simulink model "positionAlignment"  (R2019b)
settings: Solver=FixedStepAuto  StartTime=tStart  StopTime=tEnd  FixedStep=tStep  RelTol=1e-3
values from neighbouring files (symbols this model uses):
  headingCurrent = headings(ind)    [simulation.m]
  headingPrevious = -headingCurrent    [simulation.m]
  pathLength = sqrt((XYCurrent(1)-XYPrevious(1))^2 + (XYCurrent(2)-XYPrevious(2))^2)    [simulation.m]
  tStep = 0.01    [simulation.m]
  X = (1:imWidth)/imWidth*yardWidth    [getTerrainBinary1.m]
  XYCurrent = wayPointsXY(ind+1,:)    [simulation.m]
  XYPrevious = XYCurrent    [simulation.m]
  Y = (1:imHeight)/imHeight*yardHeight    [getTerrainBinary1.m]
  Z = double(yardBright)/255*height    [createVirtualWorld.m]    (also in getTerrainBinary1.m = image; getTerrainBinary2.m = image; simulation.m = (sin(4*Y))/8; terrainMain.m = getTerrainBinary2(height, yardWidth, yardHeight, yardBright,)
libraries: simulink x1
settings Model: Creator=sebas  LastModifiedBy=sebas

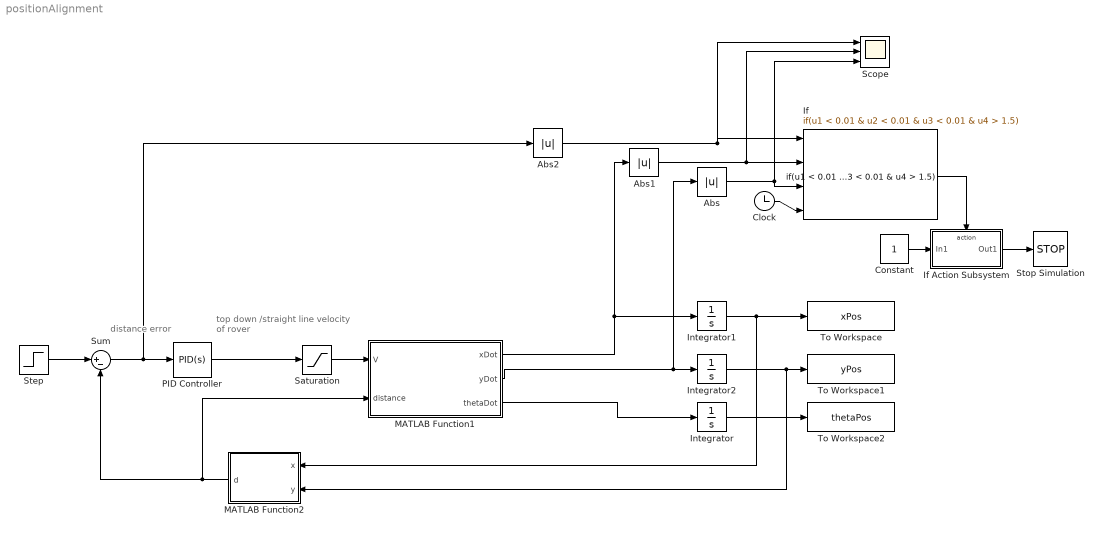
== system positionAlignment ==
  note: top down /straight line
      | velocity of rover
  note: distance error
  Abs : Abs
  Abs1 : Abs
  Abs2 : Abs
  Clock : Clock
  Constant : Constant
  If : If  NumInputs=4  IfExpression=u1 < 0.01 & u2 < 0.01 & u3 < 0.01 & u4 > 1.5  ShowElse=off
  If Action Subsystem : Subsystem  TreatAsAtomicUnit=on
  Integrator : Integrator  InitialCondition=headingPrevious
  Integrator1 : Integrator
  Integrator2 : Integrator
  MATLAB Function1 : MATLAB Function  TreatAsAtomicUnit=on
  MATLAB Function2 : MATLAB Function  TreatAsAtomicUnit=on
  PID Controller : simulink/Continuous/PID Controller  Controller=PID  Form=Parallel  TimeDomain=Continuous-time  SampleTime=-1  IntegratorMethod=Forward Euler  FilterMethod=Forward Euler  ControllerParametersSource=internal  P=0.31  I=0.0004396  D=-0.0175  UseFilter=on  N=18.11  TunerSelectOption=Transfer Function Based (PID Tuner App)  InitialConditionSource=internal  InitialConditionForIntegrator=0  InitialConditionForFilter=0  DifferentiatorICPrevScaledInput=0  ExternalReset=none  TrackingMode=off  Kt=1  LimitOutput=off  UpperSaturationLimit=inf  LowerSaturationLimit=-inf  LinearizeAsGain=on  AntiWindupMode=none  Kb=1  POutMin=[]  POutMax=[]  IOutMin=[]  IOutMax=[]  DOutMin=[]  DOutMax=[]  NOutMin=[]  NOutMax=[]  SumOutMin=[]  SumOutMax=[]  SaturationOutMin=[]  SaturationOutMax=[]  PParamMin=[]  PParamMax=[]  IParamMin=[]  IParamMax=[]  DParamMin=[]  DParamMax=[]  NParamMin=[]  NParamMax=[]  KbParamMin=[]  KbParamMax=[]  KtParamMin=[]  KtParamMax=[]  KbOutMin=[]  KbOutMax=[]  KtOutMin=[]  KtOutMax=[]  IntegratorOutMin=[]  IntegratorOutMax=[]  FilterOutMin=[]  FilterOutMax=[]  SumI1OutMin=[]  SumI1OutMax=[]  SumI2OutMin=[]  SumI2OutMax=[]  SumI3OutMin=[]  SumI3OutMax=[]  SumI4OutMin=[]  SumI4OutMax=[]  SumDOutMin=[]  SumDOutMax=[]  DifferentiatorOutMin=[]  DifferentiatorOutMax=[]  FilterDiffOutCoefMin=[]  FilterDiffOutCoefMax=[]  ReciprocalOutMin=[]  ReciprocalOutMax=[]  SumDenOutMin=[]  SumDenOutMax=[]  SumNumOutMin=[]  SumNumOutMax=[]  DivideOutMin=[]  DivideOutMax=[]  IntegratorContinuousStateAttributes=''  IntegratorStateMustResolveToSignalObject=off  IntegratorRTWStateStorageClass=Auto  FilterContinuousStateAttributes=''  FilterStateMustResolveToSignalObject=off  FilterRTWStateStorageClass=Auto  ParallelPVariant=InternalParameters  IdealPVariant=Disabled  IVariant=InternalParameters  DVariant=InternalParameters  IntegratorVariant=Continuous  SatVariant=Disabled  AWVariant=Passthrough  PCopyVariant=Disabled  TRVariant=Disabled  FdbkBlocksVariant=Forward  IdealPFdbkVariant=Disabled  SatFdbkVariant=Disabled  DerivativeFilterVariant=ContFilter  NVariant=InternalParameters  NCopyVariant=Disabled  FilterICVariant=InternalICsFilter  IntegratorICVariant=InternalICs  ExternalResetVariant=Disabled  TRSumVariant=Passthrough  SumFdbkVariant=Disabled  SumVariant=Sum_PID
  Saturation : Saturate  UpperLimit=0.05  LowerLimit=-0.05
  Scope : Scope  NumInputPorts=3
  Step : Step  Time=0  After=pathLength  SampleTime=0
  Stop Simulation : Stop
  Sum : Sum  Inputs=|+-
  To Workspace : ToWorkspace  VariableName=xPos  SaveFormat=Timeseries  SampleTime=-1
  To Workspace1 : ToWorkspace  VariableName=yPos  SaveFormat=Timeseries  SampleTime=-1
  To Workspace2 : ToWorkspace  VariableName=thetaPos  SaveFormat=Timeseries  SampleTime=-1
  wires:
  Integrator/1 -> To Workspace2/1
  PID Controller/1 -> Saturation/1
  MATLAB Function1/1(xDot) -> Abs1/1, Integrator1/1
  MATLAB Function1/3(thetaDot) -> Integrator/1
  Integrator1/1 -> To Workspace/1, MATLAB Function2/1(x)
  Step/1 -> Sum/1
  Integrator2/1 -> To Workspace1/1, MATLAB Function2/2(y)
  MATLAB Function1/2(yDot) -> Abs/1, Integrator2/1
  MATLAB Function2/1(d) -> MATLAB Function1/2(distance), Sum/2
  Saturation/1 -> MATLAB Function1/1(V)
  Constant/1 -> If Action Subsystem/1(In1)
  If Action Subsystem/1(Out1) -> Stop Simulation/1
  If/1 -> If Action Subsystem/Action
  Sum/1 -> Abs2/1, PID Controller/1
  Abs1/1 -> Scope/2, If/2
  Abs/1 -> Scope/3, If/3
  Clock/1 -> If/4
  Abs2/1 -> If/1, Scope/1

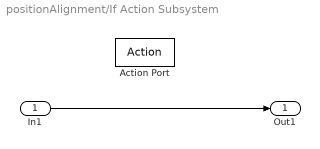
== system positionAlignment/If Action Subsystem ==
  In1 : Inport
  Action Port : ActionPort  ActionPortLabel=if(u1 < 0.1 & u2 < 0.01 & u3 < 0.01 & u4 > 1.5)
  Out1 : Outport
  wires:
  In1/1 -> Out1/1

== matlab function positionAlignment/MATLAB Function1 ==
  data: V input; distance input; xDot output; yDot output; thetaDot output; Z parameter double; XYCurrent parameter; headingCurrent parameter; XYPrevious parameter; X parameter; Y parameter; tStep parameter
function [xDot,yDot,thetaDot] = kinematical(V, distance,Z, XYCurrent, headingCurrent, XYPrevious, X, Y, tStep)




    n    = 4;                % number of wheels    (i)
    D    = 0.2286;           % diameter            (m)
    R    = D/2;              % radius              (m)
    lata = 0.5461;           % length axle to axle (m)
    wata = lata;             % width axle to axle  (m)
    ba   = [1, -1, -1, 1];   % x-wise position     (i)
    bb   = [1, 1, -1, -1];   % y-wise position     (i)


    
    newX = XYPrevious(1) + distance*sind(headingCurrent);
    newY = XYPrevious(2) + distance*cosd(headingCurrent);
    oldX = XYPrevious(1) + 0.85*distance*sind(headingCurrent);
    oldY = XYPrevious(2) + 0.85*distance*cosd(headingCurrent);
    
    
    
    % convert straight line distance covered to updated xyz
    dcm = [cosd(-headingCurrent) -sind(-headingCurrent);
        sind(-headingCurrent) cosd(-headingCurrent)];
    wheel1True = [newX; newY] + dcm*[wata/2;lata/2];
    wheel2True = [newX; newY] + dcm*[-wata/2;lata/2];
    wheel3True = [newX; newY] + dcm*[-wata/2;-lata/2];
    wheel4True = [newX; newY] + dcm*[wata/2;-lata/2];
    wheelListXY = [wheel1True';wheel2True';wheel3True';wheel4True'];
    wheelXYZ = getWaypointsElevation(wheelListXY, X, Y, Z);
    
    wheel1TruePrev = [XYPrevious(1); XYPrevious(2)] + dcm*[wata/2;lata/2];
    wheel2TruePrev = [XYPrevious(1); XYPrevious(2)] + dcm*[-wata/2;lata/2];
    wheel3TruePrev = [XYPrevious(1); XYPrevious(2)] + dcm*[-wata/2;-lata/2];
    wheel4TruePrev = [XYPrevious(1); XYPrevious(2)] + dcm*[wata/2;-lata/2];
    wheelListXYPrev = [wheel1TruePrev';wheel2TruePrev';wheel3TruePrev';wheel4TruePrev'];
    wheelXYZPrev = getWaypointsElevation(wheelListXYPrev, X, Y, Z);
    
    
    bottom = sqrt((wheelXYZ(1,1)-wheelXYZPrev(1,1))^2 + (wheelXYZ(1,2)-wheelXYZPrev(1,2))^2);
    slope = atand((wheelXYZ(1,3)-wheelXYZPrev(1,3))/bottom);
    if isnan(slope) == 1
        wheel1Slope = 0;
    else
        wheel1Slope=slope;
    end
    
    bottom = sqrt((wheelXYZ(2,1)-wheelXYZPrev(2,1))^2 + (wheelXYZ(2,2)-wheelXYZPrev(2,2))^2);
    slope = atand((wheelXYZ(2,3)-wheelXYZPrev(2,3))/bottom);
    if isnan(slope) == 1
        wheel2Slope = 0;
    else
        wheel2Slope=slope;
    end
    
    bottom = sqrt((wheelXYZ(3,1)-wheelXYZPrev(3,1))^2 + (wheelXYZ(3,2)-wheelXYZPrev(3,2))^2);
    slope = atand((wheelXYZ(3,3)-wheelXYZPrev(3,3))/bottom);
    if isnan(slope) == 1
        wheel3Slope = 0;
    else
        wheel3Slope=slope;
    end
    
    bottom = sqrt((wheelXYZ(4,1)-wheelXYZPrev(4,1))^2 + (wheelXYZ(4,2)-wheelXYZPrev(4,2))^2);
    slope = atand((wheelXYZ(4,3)-wheelXYZPrev(4,3))/bottom);
    if isnan(slope) == 1
        wheel4Slope = 0;
    else
        wheel4Slope=slope;
    end  
    
%     subplot(2,1,1)
%     axis equal
%     plot3(newX, newY, 0.5, 'bo')
%     hold on
%     plot3(wheelXYZ(:,1),wheelXYZ(:,2),wheelXYZ(:,3), 'rx', 'Linewidth', 3)

    
    
    omega = [
        V/abs(cosd(wheel1Slope));
        V/abs(cosd(wheel2Slope));
        V/abs(cosd(wheel3Slope));
        V/abs(cosd(wheel4Slope))
        ]/R;

%     figure(1)
%     subplot(2,1,2)
%     figure(2)
%     plot(omega-omega(2), 'rx')
%     hold off
%     axis([0 4 0 1])
    
    % HOMOGENOUS dimensions
    la = wata/2;    % reference to axle (X)
    lb = lata/2;    % reference to axle (Y)
    lc = la;        % reference to axle (Z)

    % WHEEL JACOBIAN (3 x 4)
    J    = (R/4)*[-1, 1, -1, 1; 1, 1, 1, 1; ...
              1/(la + lb), -1/(la + lb), -1/(la + lb), 1/(la + lb)];   

    rates = J*omega;
    xDot = rates(1);
    yDot = rates(2);
    thetaDot = rates(3);

== matlab function positionAlignment/MATLAB Function2 ==
  data: x input; d output; y input
function d = fcn(x, y)


    d = sqrt(x^2 + y^2);
